simulink model "Lab2_PartD1"  (R2025b)
settings: Solver=VariableStepAuto  StartTime=0.0  StopTime=10.0  RelTol=1e-3
settings Model: Creator=safiakhalil  LastModifiedBy=safiakhalil

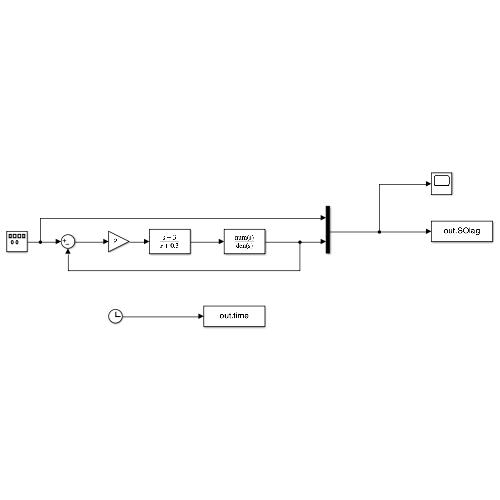
[thumbnail: Simulink's stored preview of the top-level diagram]
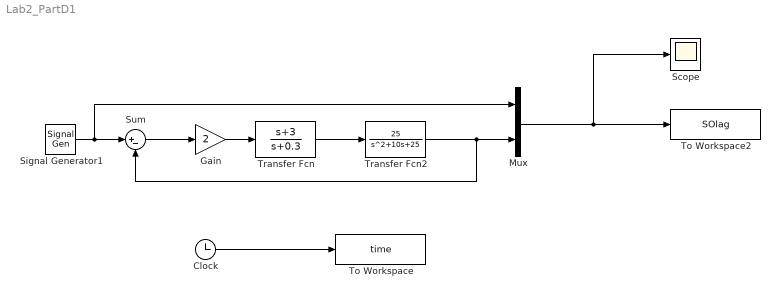
== system Lab2_PartD1 ==
  Clock : Clock
  Gain : Gain  Gain=2
  Mux : Mux  Inputs=2
  Scope : Scope
      settings: ActiveDisplayYMinimum=-1.4505162359750536  ActiveDisplayYMaximum=1.4341405617615721
  Signal Generator1 : SignalGenerator  WaveForm=square  Frequency=0.15
  Sum : Sum  Inputs=|+-
  To Workspace : ToWorkspace  VariableName=time  SampleTime=-1
  To Workspace2 : ToWorkspace  VariableName=SOlag  SampleTime=-1
  Transfer Fcn : TransferFcn  Numerator=[1 3]  Denominator=[1 0.3]
  Transfer Fcn2 : TransferFcn  Numerator=[25]  Denominator=[1 10 25]
  wires:
  Signal Generator1/1 -> Mux/1, Sum/1
  Mux/1 -> To Workspace2/1, Scope/1
  Transfer Fcn2/1 -> Sum/2, Mux/2
  Sum/1 -> Gain/1
  Gain/1 -> Transfer Fcn/1
  Transfer Fcn/1 -> Transfer Fcn2/1
  Clock/1 -> To Workspace/1
